simulink model "Practica6seminario"  (R2017b)
settings: Solver=VariableStepAuto  StartTime=0.0  StopTime=.01  RelTol=1e-3
settings Model: Creator=Charles  LastModifiedBy=Charles

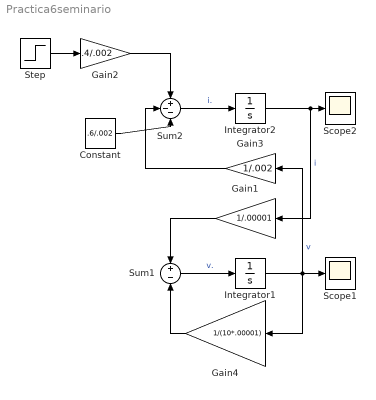
== system Practica6seminario ==
  Constant : Constant  Value=.6/.002
  Gain1 : Gain  Gain=1/.00001
  Gain2 : Gain  Gain=.4/.002
  Gain3 : Gain  Gain=1/.002
  Gain4 : Gain  Gain=1/(10*.00001)
  Integrator1 : Integrator
  Integrator2 : Integrator
  Scope1 : Scope
  Scope2 : Scope
  Step : Step  Time=0  After=32  SampleTime=0
  Sum1 : Sum  Inputs=+-
  Sum2 : Sum  Inputs=+--
  wires:
  Integrator1/1 -> Gain4/1, Gain3/1, Scope1/1  "v"
  Integrator2/1 -> Gain1/1, Scope2/1  "i"
  Step/1 -> Gain2/1
  Gain2/1 -> Sum2/1
  Sum2/1 -> Integrator2/1  "i."
  Sum1/1 -> Integrator1/1  "v."
  Gain3/1 -> Sum2/2
  Constant/1 -> Sum2/3
  Gain1/1 -> Sum1/1
  Gain4/1 -> Sum1/2
